simulink model "trjoptmz_MPC_quadcopter1"  (R2024a)
settings: Solver=VariableStepAuto  StartTime=0.0  StopTime=50  FixedStep=0.1  RelTol=1e-3
values from neighbouring files (symbols this model uses):
  g = 9.81    [Quad_innit.m]
  Iz = eye(1)    [Quad_innit.m]
  m = 2    [Quad_innit.m]
  Psi = Psi_temp    [Quad_innit.m]
  Psi_h = Psi_temp    [Quad_innit.m]
  Psi_z = Psi_temp    [Quad_innit.m]
  psid = repmat(psi,ph,1)    [Quad_innit.m]
  Theta = cat(1, Theta, Theta_row)    [Quad_innit.m]
  Theta_h = cat(1, Theta_h, Theta_row)    [Quad_innit.m]
  Theta_z = cat(1, Theta_z, Theta_row)    [Quad_innit.m]
  W3 = (W1.')*W2*W1    [Quad_innit.m]
  W3_h = (W1_h.')*W2_h*W1_h    [Quad_innit.m]
  W3_z = (W1_z.')*W2_z*W1_z    [Quad_innit.m]
  W4 = cat(1, W4, W4_row)    [Quad_innit.m]
  W4_h = cat(1, W4_h, W4_row)    [Quad_innit.m]
  W4_z = cat(1, W4_z, W4_row)    [Quad_innit.m]
libraries: slpidlib x2, sim3dlib x1, uavsim3dlib x1, uavutilslib x1
settings Model: Creator=karthikeyan  LastModifiedBy=karthikeyan

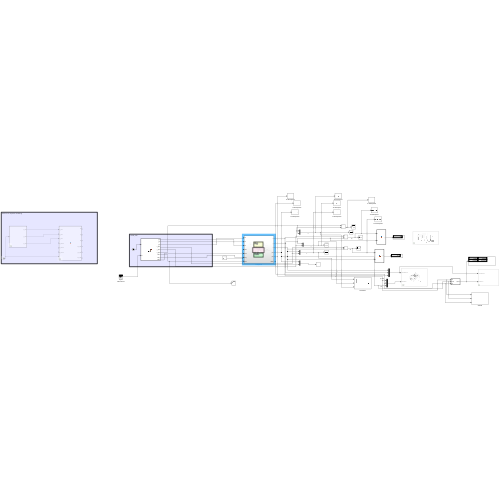
[thumbnail: Simulink's stored preview of the top-level diagram]
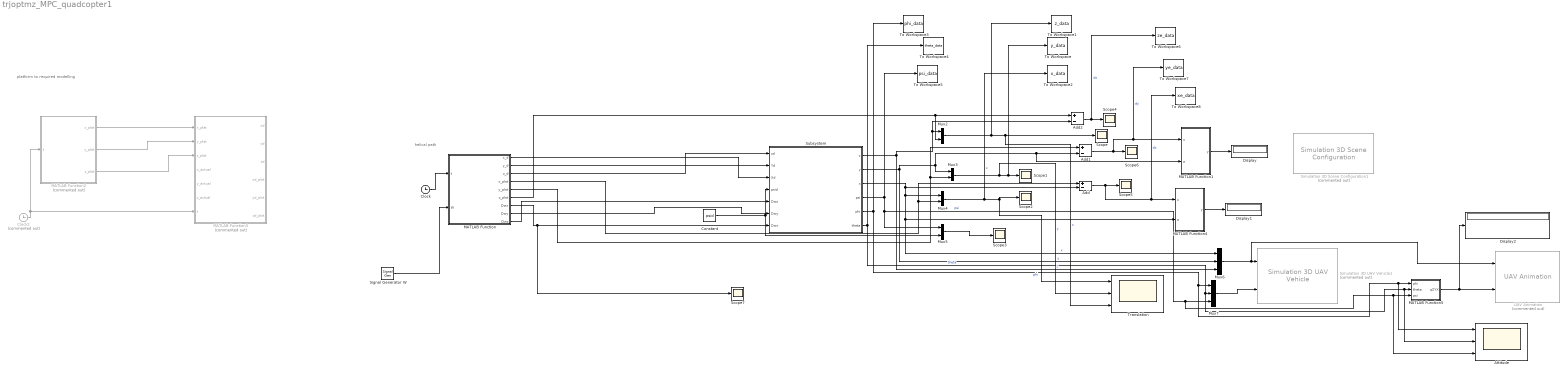
== system trjoptmz_MPC_quadcopter1 ==
  note: platform to required modelling
  note: helical path
  Add : Sum  Inputs=+-
  Add1 : Sum  Inputs=+-
  Add2 : Sum  Inputs=+-
  Attitude : Scope  NumInputPorts=3
  Clock : Clock
  Clock2 : Clock  Commented=on
  Constant : Constant  Value=psid
  Display : Display
  Display1 : Display
  Display2 : Display
  MATLAB Function : MATLAB Function  TreatAsAtomicUnit=on
  MATLAB Function1 : MATLAB Function  TreatAsAtomicUnit=on
  MATLAB Function2 : MATLAB Function  Commented=on  TreatAsAtomicUnit=on
  MATLAB Function3 : MATLAB Function  Commented=on  TreatAsAtomicUnit=on
  MATLAB Function4 : MATLAB Function  TreatAsAtomicUnit=on
  MATLAB Function5 : MATLAB Function  TreatAsAtomicUnit=on
  Mux{2..5} (4 alike) : Mux  Inputs=2
  Mux6 : Mux  Inputs=3
  Mux7 : Mux  Inputs=3
  Scope{,1..7} (8 alike) : Scope
  Signal Generator W : SignalGenerator  WaveForm=random  Units=rad/sec
  Simulation 3D Scene Configuration1 : sim3dlib/Simulation 3D Scene Configuration  Priority=0  Commented=on  ProjectFormat=Default Scenes  SceneDesc=Double lane change  ProjectName=C:\Program Files\MATLAB\R2024a\toolbox\shared\sim3d_projects\automotive_project_windows\UE\WindowsNoEditor\VehicleSimulation.exe  ScenePath=/Game/Maps/EmptyScene  EnableOpenDRIVE=off  vehTagList={'Custom';'Scene Origin';'SimulinkVehicle1';'SimulinkVehicle2'}  vehTag=SimulinkVehicle2  FreeCameraInitialTranslation=[0, 0, 0]  FreeCameraDefaultInitialTranslation=[-6, 0, 2]  FreeCameraInitialRotation=[0, 0, 0]  FreeCameraDefaultInitialRotation=[0, -15, 0]  OpVisEn=off  Ts=0.1  EnableWindow=on  EnableRemoteAccess=off  EnableWeather=off  SunAzimuth=90  SunAltitude=40.0  EnableGeospatialSun=off  Latitude=0  Longitude=0  Date=2023-01-01  Time=10:30:00  GeoTimeZone=-5.0  SunDaylightSaving=off  wind=1  clouds=10  EnableVolumetricClouds=off  CloudCoverage=0  CloudAltitude=6  fog=0  rain=0  RaindropsEffect=off  SnowDensity=0  EnableGeospatial=off  UseTrueOrigin=off  OriginHeight=200  OriginLatitude=40.744652  OriginLongitude=-73.988864  MapStyle=Aerial  AdditionalAssetIDs=[]  UseAdvancedSunSky=off  SolarTime=11  TimeZone=-5  Day=21  Month=9  Year=2022  UseDaylightSavingTime=on  DSTStartDay=10  DSTStartMonth=3  DSTEndDay=3  DSTEndMonth=11  DSTSwitchHour=2  sensorTag=MainCamera2  sensorId=2  sensorName=MainCamera2  mountLoc=Origin  offsetFlag=off  tmountOffset=[0, 0, 0]  rmountOffset=[0, 0, 0]  HorizontalResolution=1280  VerticalResolution=720  HorizontalFOV=60  mountPoint=[0 0 0]  mountOrientation=[0 0 0]  aMode=6  ID=2  GeoTrigger=Inactive
      settings: LibrarySourceBlock=robotsim3dlib/Simulation 3D Scene Configuration
  Simulation 3D UAV Vehicle1 : uavsim3dlib/Simulation 3D UAV Vehicle  Priority=-1  Commented=on  Mesh=Quadrotor  MeshPath=/MathWorksUAVContent/UAVs/HexaRotorUAV/HexaRotor.HexaRotor  Color=Black  ActorName=SimulinkVehicle2  UseGlobalFrame=off  InitialTranslation=[0 0 0]  InitialRotation=[0 0 0]  InitialTranslationGlobal=[0 0 0]  InitialGeoOrigin=[0 0 0]  InitialRotationGlobal=[0 0 0]  SampleTime=-1  ActorType=SimulinkVehicle  ID=2  aMode=4  ActorTag=SimulinkVehicle2
  Subsystem : Subsystem
  To Workspace : ToWorkspace  VariableName=y_data  SaveFormat=Structure With Time  SampleTime=-1
      settings: Save2DSignal=2-D array (concatenate along first dimension)
  To Workspace1 : ToWorkspace  VariableName=z_data  SaveFormat=Structure With Time  SampleTime=-1
      settings: Save2DSignal=2-D array (concatenate along first dimension)
  To Workspace2 : ToWorkspace  VariableName=x_data  SaveFormat=Structure With Time  SampleTime=-1
      settings: Save2DSignal=2-D array (concatenate along first dimension)
  To Workspace3 : ToWorkspace  VariableName=phi_data  SaveFormat=Structure With Time  SampleTime=-1
      settings: Save2DSignal=2-D array (concatenate along first dimension)
  To Workspace4 : ToWorkspace  VariableName=theta_data  SaveFormat=Structure With Time  SampleTime=-1
      settings: Save2DSignal=2-D array (concatenate along first dimension)
  To Workspace5 : ToWorkspace  VariableName=psi_data  SaveFormat=Structure With Time  SampleTime=-1
      settings: Save2DSignal=2-D array (concatenate along first dimension)
  To Workspace6 : ToWorkspace  VariableName=ze_data  SaveFormat=Structure With Time  SampleTime=-1
      settings: Save2DSignal=2-D array (concatenate along first dimension)
  To Workspace7 : ToWorkspace  VariableName=ye_data  SaveFormat=Structure With Time  SampleTime=-1
      settings: Save2DSignal=2-D array (concatenate along first dimension)
  To Workspace8 : ToWorkspace  VariableName=xe_data  SaveFormat=Structure With Time  SampleTime=-1
      settings: Save2DSignal=2-D array (concatenate along first dimension)
  Translation : Scope  NumInputPorts=3
  UAV Animation : uavutilslib/UAV Animation  Commented=on  UAVType=Multirotor  UAVSize=1  InertialZDirection=Up  SampleTime=-1
  wires:
  Subsystem/1(z) -> Add2/2, Mux2/1, Mux6/3  "z"
  Subsystem/2(y) -> Mux3/1, MATLAB Function1/2(a), Add1/2, Mux6/2  "y"
  Subsystem/4(psi) -> To Workspace5/1, Attitude/3, MATLAB Function5/3(psi), Mux7/3, Mux5/1  "psi"
  Mux2/1 -> To Workspace1/1, Translation/3, Scope/1  "z"
  Mux3/1 -> To Workspace/1, Scope1/1, Translation/2  "y"
  MATLAB Function2/2(y_plat) -> MATLAB Function3/2(y_plat)
  MATLAB Function2/3(z_plat) -> MATLAB Function3/3(z_plat)
  Clock2/1 -> MATLAB Function2/1(t), MATLAB Function3/7(t)
  MATLAB Function2/1(x_plat) -> MATLAB Function3/1(x_plat)
  Clock/1 -> MATLAB Function/1(t)
  MATLAB Function/1(x_d) -> Subsystem/3(Xd)
  MATLAB Function/2(y_d) -> Subsystem/2(Yd)
  MATLAB Function/3(z_d) -> Subsystem/1(zd)
  Constant/1 -> Mux5/2, Subsystem/4(psid)
  Mux4/1 -> To Workspace2/1, Scope2/1, Translation/1  "x"
  Mux5/1 -> Scope3/1
  MATLAB Function/4(x_plot) -> Add/1, Mux4/2
  MATLAB Function/5(y_plot) -> Add1/1, Mux3/2
  MATLAB Function/6(z_plot) -> Mux2/2, Add2/1
  Add2/1 -> To Workspace6/1, Scope4/1  "dz"
  Add1/1 -> Scope6/1, To Workspace7/1, MATLAB Function1/1(u)  "dy"
  MATLAB Function1/1(y) -> Display/1
  Subsystem/3(x) -> Mux6/1, MATLAB Function4/2(a), Mux4/1, Add/2  "x"
  MATLAB Function4/1(y) -> Display1/1
  Add/1 -> To Workspace8/1, MATLAB Function4/1(u), Scope5/1  "dx"
  Mux6/1 -> UAV Animation/1, Simulation 3D UAV Vehicle1/1
  Mux7/1 -> Simulation 3D UAV Vehicle1/2
  Subsystem/5(phi) -> To Workspace3/1, Attitude/1, MATLAB Function5/1(phi), Mux7/1  "phi"
  Subsystem/6(theta) -> To Workspace4/1, Attitude/2, MATLAB Function5/2(theta), Mux7/2  "theta"
  MATLAB Function5/1(qZYX) -> Display2/1, UAV Animation/2
  MATLAB Function/7(Dwx) -> Scope7/1, Subsystem/7(Dwx)
  MATLAB Function/8(Dwy) -> Subsystem/6(Dwy)
  MATLAB Function/9(Dwz) -> Subsystem/5(Dwz)
  Signal Generator W/1 -> MATLAB Function/2(W)

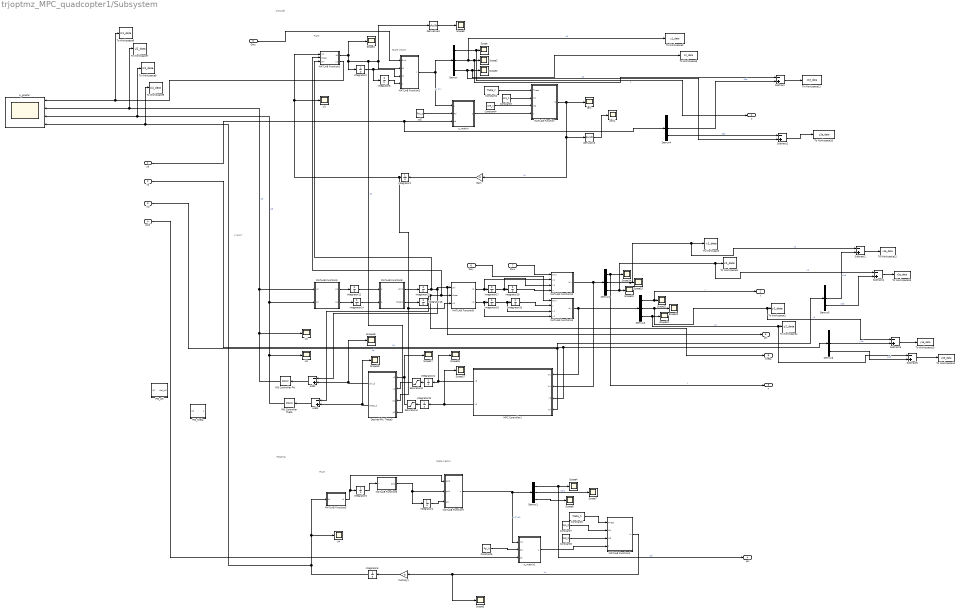
== system trjoptmz_MPC_quadcopter1/Subsystem ==
  note: X and Y
  note: Plant
  note: State Vector
  note: Altitude
  note: State Vector
  note: Plant
  note: Heading
  zd : Inport
  Yd : Inport  Port=2
  Xd : Inport  Port=3
  psid : Inport  Port=4
  Dwz : Inport  Port=5
  Dwy : Inport  Port=6
  Dwx : Inport  Port=7
  Add2 : Sum  Inputs=-+
  Add4 : Sum  Inputs=-+
  Constant2 : Constant  Value=Theta_z
  Constant3 : Constant  Value=W4_z
  Constant4 : Constant  Value=W3_z
  Constant5 : Constant  Value=Psi_h
  Constant6 : Constant  Value=Theta_h
  Constant7 : Constant  Value=W4_h
  Constant8 : Constant  Value=W3_h
  Demux{,1..6} (7 alike) : Demux  Outputs=3
  Derivative : Derivative
  Derivative1 : Derivative
  "Desired Phi, Theta3" : MATLAB Function  TreatAsAtomicUnit=on
  Gain : Gain  Gain=m
  Integrator1 : Integrator  LimitOutput=on  UpperSaturationLimit=1.5*m*g  LowerSaturationLimit=0
  Integrator{12,14..16} (4 alike) : Integrator  WrapState=on
  Integrator17 : Integrator  UpperSaturationLimit=12  LowerSaturationLimit=-12
  Integrator18 : Integrator  LowerSaturationLimit=-12
  Integrator19 : Integrator  UpperSaturationLimit=12  LowerSaturationLimit=-12
  Integrator2 : Integrator  LimitOutput=on  UpperSaturationLimit=10  LowerSaturationLimit=-10  WrappedStateUpperValue=15  WrappedStateLowerValue=-15
  Integrator20 : Integrator  UpperSaturationLimit=12  LowerSaturationLimit=-12
  Integrator21 : Integrator  UpperSaturationLimit=g  LowerSaturationLimit=-g
  Integrator22 : Integrator  UpperSaturationLimit=g  LowerSaturationLimit=-g
  Integrator3 : Integrator
  Integrator4 : Integrator
  Integrator5 : Integrator  UpperSaturationLimit=3.14  LowerSaturationLimit=-3.14  WrapState=on  WrappedStateUpperValue=0.05*1.5*m*g  WrappedStateLowerValue=-0.05*1.5*m*g
  Integrator6 : Integrator  LimitOutput=on  LowerSaturationLimit=0
  MATLAB Function : MATLAB Function  TreatAsAtomicUnit=on
  MATLAB Function1 : MATLAB Function  TreatAsAtomicUnit=on
  MATLAB Function10 : MATLAB Function  TreatAsAtomicUnit=on
  MATLAB Function11 : MATLAB Function  TreatAsAtomicUnit=on
  MATLAB Function2 : MATLAB Function  TreatAsAtomicUnit=on
  MATLAB Function3 : MATLAB Function  TreatAsAtomicUnit=on
  MATLAB Function4 : MATLAB Function  TreatAsAtomicUnit=on
  MATLAB Function5 : MATLAB Function  TreatAsAtomicUnit=on
  MATLAB Function6 : MATLAB Function  TreatAsAtomicUnit=on
  MATLAB Function7 : MATLAB Function  TreatAsAtomicUnit=on
  MATLAB Function8 : MATLAB Function  TreatAsAtomicUnit=on
  MATLAB Function9 : MATLAB Function  TreatAsAtomicUnit=on
  MPC Controller1 : Subsystem
  Multiply1 : Gain  Gain=Iz
  PID Controller Phi : slpidlib/PID Controller  Controller=PID  Form=Parallel  TimeDomain=Continuous-time  UseExternalTs=off  SampleTime=-1  IntegratorMethod=Forward Euler  FilterMethod=Forward Euler  ControllerParametersSource=internal  P=9931.26258398968  I=92443.4670455248  UseKiTs=off  D=250  UseExternalDerivativeSource=off  N=24410.9463918725  UseFilter=on  TunerSelectOption=Transfer Function Based (PID Tuner App)  InitialConditionSource=internal  InitialConditionForIntegrator=0  InitialConditionForFilter=0  DifferentiatorICPrevScaledInput=0  ExternalReset=none  TrackingMode=off  Kt=1  LimitOutput=off  SatLimitsSource=internal  UpperSaturationLimit=inf  LowerSaturationLimit=-inf  LinearizeAsGain=on  AntiWindupMode=none  Kb=1  LimitIntegrator=off  UpperIntegratorSaturationLimit=inf  LowerIntegratorSaturationLimit=-inf  POutMin=[]  POutMax=[]  IOutMin=[]  IOutMax=[]  DOutMin=[]  DOutMax=[]  NOutMin=[]  NOutMax=[]  SumOutMin=[]  SumOutMax=[]  SaturationOutMin=[]  SaturationOutMax=[]  PParamMin=[]  PParamMax=[]  IParamMin=[]  IParamMax=[]  DParamMin=[]  DParamMax=[]  NParamMin=[]  NParamMax=[]  KbParamMin=[]  KbParamMax=[]  KtParamMin=[]  KtParamMax=[]  KbOutMin=[]  KbOutMax=[]  KtOutMin=[]  KtOutMax=[]  IntegratorOutMin=[]  IntegratorOutMax=[]  FilterOutMin=[]  FilterOutMax=[]  SumI1OutMin=[]  SumI1OutMax=[]  SumI2OutMin=[]  SumI2OutMax=[]  SumI3OutMin=[]  SumI3OutMax=[]  SumI4OutMin=[]  SumI4OutMax=[]  SumDOutMin=[]  SumDOutMax=[]  DifferentiatorOutMin=[]  DifferentiatorOutMax=[]  FilterDiffOutCoefMin=[]  FilterDiffOutCoefMax=[]  ReciprocalOutMin=[]  ReciprocalOutMax=[]  SumDenOutMin=[]  SumDenOutMax=[]  SumNumOutMin=[]  SumNumOutMax=[]  DivideOutMin=[]  DivideOutMax=[]  UdiffTsProdOutMin=[]  UdiffTsProdOutMax=[]  NTsProdOutMin=[]  NTsProdOutMax=[]  UintegralTsProdOutMin=[]  UintegralTsProdOutMax=[]  UngainTsProdOutMin=[]  UngainTsProdOutMax=[]  ClampingZeroOutDataTypeStr=Inherit: Inherit via back propagation  ClampingZeroOutMin=[]  ClampingZeroOutMax=[]  FilterDenConstantOutDataTypeStr=Inherit: Inherit via back propagation  FilterDenConstantOutMin=[]  FilterDenConstantOutMax=[]  PCopyOutDataTypeStr=Inherit: Inherit via back propagation  PCopyOutMin=[]  PCopyOutMax=[]  NCopyOutDataTypeStr=Inherit: Inherit via back propagation  NCopyOutMin=[]  NCopyOutMax=[]  IntegratorContinuousStateAttributes=''  IntegratorStateMustResolveToSignalObject=off  IntegratorRTWStateStorageClass=Auto  FilterContinuousStateAttributes=''  FilterStateMustResolveToSignalObject=off  FilterRTWStateStorageClass=Auto  ParallelPVariant=InternalParameters  IdealPVariant=Disabled  IVariant=InternalParameters  DVariant=InternalParameters  IntegratorVariant=Continuous  SatVariant=Disabled  AWVariant=Passthrough  PCopyVariant=Disabled  TRVariant=Disabled  FdbkBlocksVariant=Forward  IdealPFdbkVariant=Disabled  SatFdbkVariant=Disabled  DerivativeFilterVariant=ContFilter  NVariant=InternalParameters  NCopyVariant=Disabled  FilterICVariant=InternalICsFilter  IntegratorICVariant=InternalICs  ExternalResetVariant=Disabled  TRSumVariant=Passthrough  SumFdbkVariant=Disabled  SumVariant=Sum_PID  TsampFilterVariant=InternalTs  TsampNgainVariant=Passthrough  TsampIntegralVariant=Disabled_SignalSpec  ExternalSaturationOutDataTypeStr=Inherit: Same as second input  DerivativeSourceVariant=ErrorSignal
  PID Controller Theta : slpidlib/PID Controller  Controller=PID  Form=Parallel  TimeDomain=Continuous-time  UseExternalTs=off  SampleTime=-1  IntegratorMethod=Forward Euler  FilterMethod=Forward Euler  ControllerParametersSource=internal  P=10811.4487421448  I=110533.695685683  UseKiTs=off  D=250  UseExternalDerivativeSource=off  N=24410.9463914125  UseFilter=on  TunerSelectOption=Transfer Function Based (PID Tuner App)  InitialConditionSource=internal  InitialConditionForIntegrator=0  InitialConditionForFilter=0  DifferentiatorICPrevScaledInput=0  ExternalReset=none  TrackingMode=off  Kt=1  LimitOutput=off  SatLimitsSource=internal  UpperSaturationLimit=inf  LowerSaturationLimit=-inf  LinearizeAsGain=on  AntiWindupMode=none  Kb=1  LimitIntegrator=off  UpperIntegratorSaturationLimit=inf  LowerIntegratorSaturationLimit=-inf  POutMin=[]  POutMax=[]  IOutMin=[]  IOutMax=[]  DOutMin=[]  DOutMax=[]  NOutMin=[]  NOutMax=[]  SumOutMin=[]  SumOutMax=[]  SaturationOutMin=[]  SaturationOutMax=[]  PParamMin=[]  PParamMax=[]  IParamMin=[]  IParamMax=[]  DParamMin=[]  DParamMax=[]  NParamMin=[]  NParamMax=[]  KbParamMin=[]  KbParamMax=[]  KtParamMin=[]  KtParamMax=[]  KbOutMin=[]  KbOutMax=[]  KtOutMin=[]  KtOutMax=[]  IntegratorOutMin=[]  IntegratorOutMax=[]  FilterOutMin=[]  FilterOutMax=[]  SumI1OutMin=[]  SumI1OutMax=[]  SumI2OutMin=[]  SumI2OutMax=[]  SumI3OutMin=[]  SumI3OutMax=[]  SumI4OutMin=[]  SumI4OutMax=[]  SumDOutMin=[]  SumDOutMax=[]  DifferentiatorOutMin=[]  DifferentiatorOutMax=[]  FilterDiffOutCoefMin=[]  FilterDiffOutCoefMax=[]  ReciprocalOutMin=[]  ReciprocalOutMax=[]  SumDenOutMin=[]  SumDenOutMax=[]  SumNumOutMin=[]  SumNumOutMax=[]  DivideOutMin=[]  DivideOutMax=[]  UdiffTsProdOutMin=[]  UdiffTsProdOutMax=[]  NTsProdOutMin=[]  NTsProdOutMax=[]  UintegralTsProdOutMin=[]  UintegralTsProdOutMax=[]  UngainTsProdOutMin=[]  UngainTsProdOutMax=[]  ClampingZeroOutDataTypeStr=Inherit: Inherit via back propagation  ClampingZeroOutMin=[]  ClampingZeroOutMax=[]  FilterDenConstantOutDataTypeStr=Inherit: Inherit via back propagation  FilterDenConstantOutMin=[]  FilterDenConstantOutMax=[]  PCopyOutDataTypeStr=Inherit: Inherit via back propagation  PCopyOutMin=[]  PCopyOutMax=[]  NCopyOutDataTypeStr=Inherit: Inherit via back propagation  NCopyOutMin=[]  NCopyOutMax=[]  IntegratorContinuousStateAttributes=''  IntegratorStateMustResolveToSignalObject=off  IntegratorRTWStateStorageClass=Auto  FilterContinuousStateAttributes=''  FilterStateMustResolveToSignalObject=off  FilterRTWStateStorageClass=Auto  ParallelPVariant=InternalParameters  IdealPVariant=Disabled  IVariant=InternalParameters  DVariant=InternalParameters  IntegratorVariant=Continuous  SatVariant=Disabled  AWVariant=Passthrough  PCopyVariant=Disabled  TRVariant=Disabled  FdbkBlocksVariant=Forward  IdealPFdbkVariant=Disabled  SatFdbkVariant=Disabled  DerivativeFilterVariant=ContFilter  NVariant=InternalParameters  NCopyVariant=Disabled  FilterICVariant=InternalICsFilter  IntegratorICVariant=InternalICs  ExternalResetVariant=Disabled  TRSumVariant=Passthrough  SumFdbkVariant=Disabled  SumVariant=Sum_PID  TsampFilterVariant=InternalTs  TsampNgainVariant=Passthrough  TsampIntegralVariant=Disabled_SignalSpec  ExternalSaturationOutDataTypeStr=Inherit: Same as second input  DerivativeSourceVariant=ErrorSignal
  PID_phi : Subsystem
  PID_theta : Subsystem
  Saturation3 : Saturate  UpperLimit=1  LowerLimit=-1
  Saturation4 : Saturate  UpperLimit=1  LowerLimit=-1
  Scope{,1..5,7..9,14..15,17..23,26..27} (20 alike) : Scope
  Subtract{,1..5} (6 alike) : Sum  Inputs=-+
  To Workspace : ToWorkspace  VariableName=x1_data  SaveFormat=Structure With Time  SampleTime=-1
      settings: Save2DSignal=2-D array (concatenate along first dimension)
  To Workspace1 : ToWorkspace  VariableName=y1_data  SaveFormat=Structure With Time  SampleTime=-1
      settings: Save2DSignal=2-D array (concatenate along first dimension)
  To Workspace10 : ToWorkspace  VariableName=z2e_data  SaveFormat=Structure With Time  SampleTime=-1
      settings: Save2DSignal=2-D array (concatenate along first dimension)
  To Workspace11 : ToWorkspace  VariableName=z1e_data  SaveFormat=Structure With Time  SampleTime=-1
      settings: Save2DSignal=2-D array (concatenate along first dimension)
  To Workspace12 : ToWorkspace  VariableName=x1e_data  SaveFormat=Structure With Time  SampleTime=-1
      settings: Save2DSignal=2-D array (concatenate along first dimension)
  To Workspace13 : ToWorkspace  VariableName=x2e_data  SaveFormat=Structure With Time  SampleTime=-1
      settings: Save2DSignal=2-D array (concatenate along first dimension)
  To Workspace14 : ToWorkspace  VariableName=y2e_data  SaveFormat=Structure With Time  SampleTime=-1
      settings: Save2DSignal=2-D array (concatenate along first dimension)
  To Workspace15 : ToWorkspace  VariableName=y1e_data  SaveFormat=Structure With Time  SampleTime=-1
      settings: Save2DSignal=2-D array (concatenate along first dimension)
  To Workspace2 : ToWorkspace  VariableName=z1_data  SaveFormat=Structure With Time  SampleTime=-1
      settings: Save2DSignal=2-D array (concatenate along first dimension)
  To Workspace3 : ToWorkspace  VariableName=x2_data  SaveFormat=Structure With Time  SampleTime=-1
      settings: Save2DSignal=2-D array (concatenate along first dimension)
  To Workspace4 : ToWorkspace  VariableName=y2_data  SaveFormat=Structure With Time  SampleTime=-1
      settings: Save2DSignal=2-D array (concatenate along first dimension)
  To Workspace5 : ToWorkspace  VariableName=z2_data  SaveFormat=Structure With Time  SampleTime=-1
      settings: Save2DSignal=2-D array (concatenate along first dimension)
  To Workspace6 : ToWorkspace  VariableName=U1_data  SaveFormat=Structure With Time  SampleTime=-1
      settings: Save2DSignal=2-D array (concatenate along first dimension)
  To Workspace7 : ToWorkspace  VariableName=U2_data  SaveFormat=Structure With Time  SampleTime=-1
      settings: Save2DSignal=2-D array (concatenate along first dimension)
  To Workspace8 : ToWorkspace  VariableName=U3_data  SaveFormat=Structure With Time  SampleTime=-1
      settings: Save2DSignal=2-D array (concatenate along first dimension)
  To Workspace9 : ToWorkspace  VariableName=U4_data  SaveFormat=Structure With Time  SampleTime=-1
      settings: Save2DSignal=2-D array (concatenate along first dimension)
  U{1..4} (4 alike) : Scope
  U_graphs : Scope  NumInputPorts=4
  jerk : Scope
  jerk1 : Scope
  s_matrix : MATLAB Function  TreatAsAtomicUnit=on
  s_matrix1 : MATLAB Function  TreatAsAtomicUnit=on
  zd2 : Constant  Value=Psi_z
  z : Outport
  y : Outport  Port=2
  x : Outport  Port=3
  psi : Outport  Port=4
  phi : Outport  Port=5
  theta : Outport  Port=6
  wires:
  Integrator3/1 -> MATLAB Function6/1(r)
  Integrator14/1 -> MATLAB Function8/2(q)
  MATLAB Function3/2(q1) -> Integrator14/1
  Derivative1/1 -> Scope9/1
  PID Controller Phi/1 -> To Workspace7/1, U_graphs/2, MATLAB Function3/1(u2), U2/1  "U2"
  Integrator4/1 -> MATLAB Function7/3(psi)
  Integrator6/1 -> MATLAB Function2/4(z)
  Demux2/1 -> x/1, Scope14/1  "x"
  "Desired Phi, Theta3"/1(phi_d) -> Add2/2, Scope18/1
  Integrator19/1 -> MATLAB Function10/4(x)
  Multiply1/1 -> Integrator5/1
  Integrator16/1 -> Add4/1, theta/1, MATLAB Function1/2(theta), MATLAB Function9/2(theta)
  Demux1/1 -> psi/1, Scope4/1  "psi"
  MATLAB Function1/1(z2) -> "Desired Phi, Theta3"/4(z2), Derivative1/1, MATLAB Function2/2(z2), Integrator2/1, Scope1/1  "z2"
  Constant3/1 -> MATLAB Function/2(W4)
  Integrator2/1 -> MATLAB Function2/3(z1), Integrator6/1
  Demux/3 -> Subtract1/2, To Workspace5/1, Scope3/1  "z2"
  MATLAB Function6/1(psi1) -> Integrator4/1, MATLAB Function7/2(psi1)
  Add4/1 -> PID Controller Theta/1
  Demux3/1 -> y/1, Scope21/1  "y"
  MATLAB Function4/1(vk) -> Scope5/1, Multiply1/1  "Vk"
  Integrator5/1 -> To Workspace9/1, U_graphs/4, MATLAB Function5/1(U4), U4/1
  s_matrix/1(s) -> MATLAB Function/4(s)
  Integrator17/1 -> MATLAB Function10/3(x1), Integrator19/1
  Integrator21/1 -> Saturation3/1
  Integrator15/1 -> MATLAB Function1/3(phi), Add2/1, phi/1, MATLAB Function9/1(phi)
  MATLAB Function/1(vk) -> Gain/1, Derivative/1, jerk/1  "Vk"
  Gain/1 -> Integrator1/1
  MATLAB Function5/1(r1) -> Integrator3/1, MATLAB Function7/1(psi2)
  Add2/1 -> PID Controller Phi/1
  Demux/1 -> z/1, Scope/1  "z"
  PID Controller Theta/1 -> To Workspace8/1, U_graphs/3, MATLAB Function3/2(u3), U3/1  "U3"
  MATLAB Function7/1(w) -> Demux1/1, s_matrix1/1(Wk)  "z = Wk"
  Integrator18/1 -> MATLAB Function11/3(y1), Integrator20/1
  zd2/1 -> s_matrix/2(Psi)
  MATLAB Function9/2(y2) -> MATLAB Function11/4(y2), Integrator18/1
  Integrator1/1 -> MATLAB Function9/3(U1), "Desired Phi, Theta3"/3(U1), MATLAB Function1/1(U1), U1/1
  "Desired Phi, Theta3"/2(theta_d) -> Scope19/1, Add4/2
  Derivative/1 -> jerk1/1
  Constant2/1 -> MATLAB Function/1(Theta)
  Saturation4/1 -> Scope17/1, "Desired Phi, Theta3"/1(x2)
  Constant7/1 -> MATLAB Function4/2(W4)
  Constant5/1 -> s_matrix1/2(Psi)
  Integrator20/1 -> MATLAB Function11/2(y)
  Constant8/1 -> MATLAB Function4/3(W3)
  Demux1/3 -> Scope8/1
  Demux2/3 -> Subtract4/1, To Workspace3/1, Scope20/1  "x2"
  psid/1 -> s_matrix1/3(zd)
  Demux2/2 -> Subtract2/1, To Workspace/1, Scope15/1  "x1"
  Demux1/2 -> Scope7/1  "psi1"
  Constant4/1 -> MATLAB Function/3(W3)
  MATLAB Function3/1(p1) -> Integrator12/1
  MATLAB Function8/2(theta1) -> Integrator16/1
  Demux/2 -> To Workspace2/1, Subtract/1, Scope2/1  "z1"
  MATLAB Function10/1(Wx) -> Demux2/1, MPC Controller1/2(Wx)
  MATLAB Function8/1(phi1) -> Integrator15/1
  Demux3/2 -> Subtract3/1, To Workspace1/1, Scope22/1  "y1"
  Demux3/3 -> Subtract5/1, To Workspace4/1, Scope23/1  "y2"
  MATLAB Function11/1(Wy) -> MPC Controller1/1(Wy), Demux3/1
  Integrator12/1 -> MATLAB Function8/1(p)
  MPC Controller1/1(y3) -> Integrator21/1, Scope26/1
  MATLAB Function2/1(x) -> s_matrix/1(x), Demux/1  "y = x"
  MATLAB Function9/1(x2) -> MATLAB Function10/2(x2), Integrator17/1
  MPC Controller1/2(x3) -> Scope27/1, Integrator22/1
  Saturation3/1 -> "Desired Phi, Theta3"/2(y2)
  Integrator22/1 -> Saturation4/1
  Constant6/1 -> MATLAB Function4/1(Theta)
  s_matrix1/1(s) -> MATLAB Function4/4(s)
  Xd/1 -> Demux5/1, MPC Controller1/4(Xd)  "Xd"
  zd/1 -> Demux4/1, s_matrix/3(zd)
  Yd/1 -> Demux6/1, MPC Controller1/3(Yd)  "Yd"
  MATLAB Function1/2(u1) -> To Workspace6/1, U_graphs/1
  Dwz/1 -> MATLAB Function2/1(Dwz)
  Dwx/1 -> MATLAB Function10/1(Dwx)
  Dwy/1 -> MATLAB Function11/1(Dwx)
  Demux4/2 -> Subtract/2  "z1d"
  Demux4/3 -> Subtract1/1  "z2d"
  Subtract/1 -> To Workspace11/1
  Subtract1/1 -> To Workspace10/1
  Demux5/2 -> Subtract2/2  "x1d"
  Demux5/3 -> Subtract4/2  "x2d"
  Demux6/2 -> Subtract3/2  "y1d"
  Demux6/3 -> Subtract5/2  "y2d"
  Subtract2/1 -> To Workspace12/1
  Subtract4/1 -> To Workspace13/1
  Subtract5/1 -> To Workspace14/1
  Subtract3/1 -> To Workspace15/1

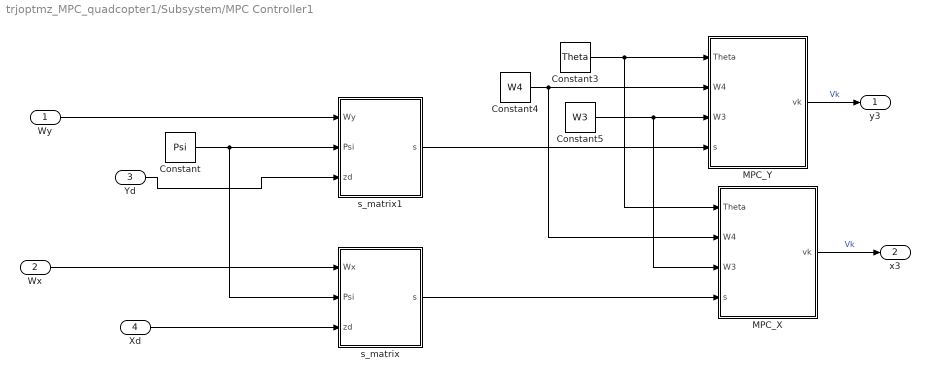
== system trjoptmz_MPC_quadcopter1/Subsystem/MPC Controller1 ==
  Wy : Inport
  Wx : Inport  Port=2
  Yd : Inport  Port=3
  Xd : Inport  Port=4
  Constant : Constant  Value=Psi
  Constant3 : Constant  Value=Theta
  Constant4 : Constant  Value=W4
  Constant5 : Constant  Value=W3
  MPC_X : MATLAB Function  TreatAsAtomicUnit=on
  MPC_Y : MATLAB Function  TreatAsAtomicUnit=on
  s_matrix : MATLAB Function  TreatAsAtomicUnit=on
  s_matrix1 : MATLAB Function  TreatAsAtomicUnit=on
  y3 : Outport
  x3 : Outport  Port=2
  wires:
  Constant3/1 -> MPC_Y/1(Theta), MPC_X/1(Theta)
  Constant/1 -> s_matrix1/2(Psi), s_matrix/2(Psi)
  Constant4/1 -> MPC_Y/2(W4), MPC_X/2(W4)
  Constant5/1 -> MPC_Y/3(W3), MPC_X/3(W3)
  s_matrix1/1(s) -> MPC_Y/4(s)
  s_matrix/1(s) -> MPC_X/4(s)
  Xd/1 -> s_matrix/3(zd)
  Yd/1 -> s_matrix1/3(zd)
  MPC_Y/1(vk) -> y3/1  "Vk"
  MPC_X/1(vk) -> x3/1  "Vk"
  Wx/1 -> s_matrix/1(Wx)
  Wy/1 -> s_matrix1/1(Wy)

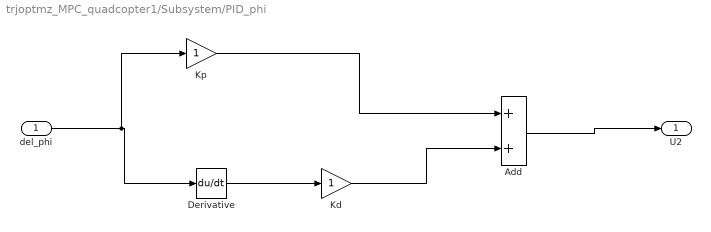
== system trjoptmz_MPC_quadcopter1/Subsystem/PID_phi ==
  del_phi : Inport
  Add : Sum
  Derivative : Derivative
  Kd : Gain
  Kp : Gain
  U2 : Outport
  wires:
  del_phi/1 -> Derivative/1, Kp/1
  Derivative/1 -> Kd/1
  Kp/1 -> Add/1
  Add/1 -> U2/1
  Kd/1 -> Add/2

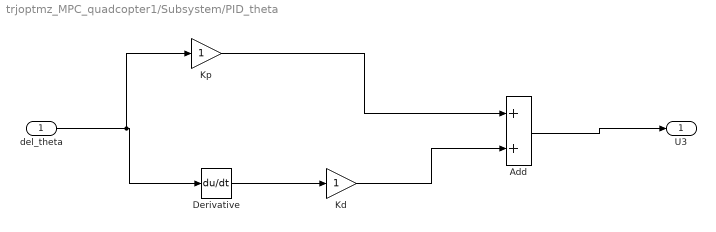
== system trjoptmz_MPC_quadcopter1/Subsystem/PID_theta ==
  del_theta : Inport
  Add : Sum
  Derivative : Derivative
  Kd : Gain
  Kp : Gain
  U3 : Outport
  wires:
  del_theta/1 -> Derivative/1, Kp/1
  Derivative/1 -> Kd/1
  Kp/1 -> Add/1
  Add/1 -> U3/1
  Kd/1 -> Add/2

== matlab function trjoptmz_MPC_quadcopter1/Subsystem/s_matrix1 ==
  data: Wk input; Psi input; zd input; s output
function s = fcn(Wk,Psi,zd)
% zk = C1*Wk;
s = zd-(Psi*Wk);

== matlab function trjoptmz_MPC_quadcopter1/MATLAB Function ==
  data: t input; x_d output; y_d output; z_d output; x_plot output; y_plot output; z_plot output; Dwx output; Dwy output; Dwz output; W input
function [x_d, y_d, z_d, x_plot, y_plot, z_plot, Dwx, Dwy, Dwz]= trajectory(t,W)


R = 2;
w = 0.1*3.14;
p = 5;
pz = 5;
h = 0.5;
del_t = 0.01;
%% Circular spiral Trajectory
% x_func = @(u) R*sin(u*w);
% y_func = @(u) R - r(u)*cos(u*w);
% z_func = @(u) 0.5*u;
% 
% x_v_func = @(u) R*w*(cos(u*w));
% y_v_func = @(u) R*w*(sin(u*w));
% z_v_func = @(u) 0.5;
% 
% x_a_func = @(u) -R*w^2 *(sin(u*w));%-r*w^2 *sin(u*w);
% y_a_func = @(u) R*w^2 *(cos(u*w));
% z_a_func = @(u) 0;

%% Conical spiral Trajectory
r = @(u) u*pi/100;
x_func = @(u) r(u)*cos(u*w);
y_func = @(u) r(u)*sin(u*w);
z_func = @(u) 0.5*u;

x_v_func = @(u) -r(u)*w*(sin(u*w));
y_v_func = @(u) r(u)*w*(cos(u*w));
z_v_func = @(u) 0.5;

x_a_func = @(u) -r(u)*w^2 *(cos(u*w));%-r*w^2 *sin(u*w);
y_a_func = @(u) -r(u)*w^2 *(sin(u*w));
z_a_func = @(u) 0;
%% Climb and track 8


dwx =@(u) (2*sin(W*pi*u));
dwy =@(u) -1*sin(W*pi*u);
dwz =@(u) 0.8*sin(W*pi*u);

xd = zeros(p*3, 1);
yd = zeros(p*3, 1);
zd = zeros(p*3, 1);


flag = 1;
for i = 0:p-1
    xd(flag) = x_func(t + i*del_t);
    xd(flag + 1) = x_v_func(t + i*del_t);
    xd(flag + 2) = x_a_func(t+ i*del_t);

    yd(flag ) = y_func(t+ i*del_t);
    yd(flag + 1) = y_v_func(t+ i*del_t);
    yd(flag +2) = y_a_func(t+ i*del_t);

    zd(flag  ) = z_func(t+ i*del_t);
    zd(flag + 1) = z_v_func(t+ i*del_t);
    zd(flag + 2) = z_a_func(t+ i*del_t);

    flag = flag + 3;


end

x_d = xd;
y_d = yd;
z_d = zd;

x_plot = xd(1);
y_plot = yd(1);
z_plot = zd(1);

Dwx = 0; %dwx(t);
Dwy = 0; %dwy(t);
Dwz = 0; %dwz(t);

== matlab function trjoptmz_MPC_quadcopter1/MATLAB Function2 ==
  data: t input; x_plat output; y_plat output; z_plat output
function [x_plat, y_plat, z_plat] = platform_trajectory(t)





r = 5;
w = 3;


x_plat = 3;
y_plat = 4;
z_plat = 0;

== matlab function trjoptmz_MPC_quadcopter1/Subsystem/Desired Phi, Theta3 ==
  data: x2 input; phi_d output; y2 input; theta_d output; U1 input; z2 input
function [phi_d,theta_d] = fcn(x2,y2,U1,z2)
m = 2; g = 9.81; 
U1 = m*g; z2 = 0; % Hover condition
if U1 == 0
    U1 = 1e-3;
end
if z2 == -g
    z2 = z2+(1e-3);
end
theta_d = asin((-m*x2/U1));
phi_d = atan(cos(theta_d)*y2/(z2+g));

== matlab function trjoptmz_MPC_quadcopter1/Subsystem/MATLAB Function3 ==
  data: u2 input; p1 output; u3 input; q1 output
function [p1,q1] = fcn(u2,u3)
Ix = 1.25; Iy = 1.25;

p1 = u2/Ix;
q1 = u3/Iy;

== matlab function trjoptmz_MPC_quadcopter1/Subsystem/MATLAB Function8 ==
  data: p input; phi1 output; q input; theta1 output
function [phi1,theta1] = fcn(p,q)

phi1 = p;
theta1 = q;

== matlab function trjoptmz_MPC_quadcopter1/Subsystem/MATLAB Function9 ==
  data: phi input; x2 output; theta input; y2 output; U1 input
function [x2,y2] = fcn(phi,theta,U1)
m = 2; g = 9.81;
%U1 = m*g;  % Hover condition

x2 = -sin(theta)*U1/m;
y2 = sin(phi)*cos(theta)*U1/m;

== matlab function trjoptmz_MPC_quadcopter1/Subsystem/MATLAB Function10 ==
  data: Dwx input; x2 input; x1 input; x input; Wx output
function Wx = fcn(Dwx,x2,x1,x)

Wx = [x;x1;(x2+Dwx)];

== matlab function trjoptmz_MPC_quadcopter1/Subsystem/MATLAB Function11 ==
  data: Dwx input; y input; Wy output; y1 input; y2 input
function Wy = fcn(Dwx,y,y1,y2)

Wy = [y;y1;(y2+Dwx)];

== matlab function trjoptmz_MPC_quadcopter1/Subsystem/MPC Controller1/MPC_X ==
  data: Theta input; vk output; W4 input; W3 input; s input
function vk = fcn(Theta,W4,W3,s)
T = Theta.';

v = (inv((T*W4*Theta)+W3))*(T)*W4*s;
vk = v(1);

== matlab function trjoptmz_MPC_quadcopter1/Subsystem/MPC Controller1/MPC_Y ==
  data: Theta input; vk output; W4 input; W3 input; s input
function vk = fcn(Theta,W4,W3,s)
T = Theta.';

v = (inv((T*W4*Theta)+W3))*(T)*W4*s;
vk = v(1);

== matlab function trjoptmz_MPC_quadcopter1/Subsystem/MPC Controller1/s_matrix ==
  data: Wx input; Psi input; zd input; s output
function s = fcn(Wx,Psi,zd)

s = zd-(Psi*Wx);

== matlab function trjoptmz_MPC_quadcopter1/Subsystem/MPC Controller1/s_matrix1 ==
  data: Wy input; Psi input; zd input; s output
function s = fcn(Wy,Psi,zd)

s = zd-(Psi*Wy);

== matlab function trjoptmz_MPC_quadcopter1/Subsystem/MATLAB Function ==
  data: Theta input; vk output; W4 input; W3 input; s input
function vk = fcn(Theta,W4,W3,s)
T = Theta.';

v = (inv((T*W4*Theta)+W3))*(T)*W4*s;
vk = v(1);

== matlab function trjoptmz_MPC_quadcopter1/MATLAB Function3 ==
  data: x_plat input; xd output; yd output; zd output; y_plat input; z_plat input; xd_plot output; yd_plot output; zd_plot output; x_actual input; y_actual input; z_actual input; t input
function [xd, yd, zd, xd_plot, yd_plot, zd_plot] = trajectory(x_plat,y_plat,z_plat, x_actual, y_actual, z_actual, t)


p = 5;
h = 0.1;


if z_actual <= 10
    zd = repmat([10; 0 ; 0], p, 1);
    xd = repmat([x_actual; 0 ; 0], p , 1);
    yd = repmat([y_actual; 0 ; 0], p, 1);

    if((x_plat - x_actual) < ERROR && (y_plat - y_actual) < ERROR)
    
    z_traj = 0;
    zd = repmat([z_traj; 0 ; 0], p, 1);
    else
    xd = repmat([x_plat; 0 ; 0], p, 1);
    yd = repmat([y_plat; 0;0], p, 1);

    end
else
    zd = repmat([10; 0 ; 0], p, 1);
    xd = repmat([x_plat; 0 ; 0], p , 1);
    yd = repmat([y_plat; 0 ; 0], p, 1);
end 



zd_plot = zd(1);
yd_plot = yd(1);
xd_plot = xd(1);

== matlab function trjoptmz_MPC_quadcopter1/MATLAB Function1 ==
  data: u input; y output; a input
function y = fcn(u,a)

y = u*100/a;

== matlab function trjoptmz_MPC_quadcopter1/MATLAB Function4 ==
  data: u input; y output; a input
function y = fcn(u,a)

y = u*100/a;

== matlab function trjoptmz_MPC_quadcopter1/Subsystem/s_matrix ==
  data: x input; Psi input; zd input; s output
function s = fcn(x,Psi,zd)

s = zd-(Psi*x);

== matlab function trjoptmz_MPC_quadcopter1/Subsystem/MATLAB Function1 ==
  data: U1 input; z2 output; theta input; phi input; u1 output
function [z2,u1] = fcn(U1,theta, phi)

%phi = 0; theta = 0; 
g = 9.81; m = 2;
u1 = U1/(cos(phi)*cos(theta));
z2 = (cos(phi)*cos(theta)*u1/m)-g;

== matlab function trjoptmz_MPC_quadcopter1/Subsystem/MATLAB Function2 ==
  data: Dwz input; z2 input; x output; z1 input; z input
function x = fcn(Dwz,z2,z1,z)

x = [z;z1;(z2+Dwz)];

== matlab function trjoptmz_MPC_quadcopter1/MATLAB Function5 ==
  data: phi input; qZYX output; theta input; psi input
function qZYX = fcn(phi,theta,psi)

eul = [psi theta phi];
qZYX = eul2quat(eul);

== matlab function trjoptmz_MPC_quadcopter1/Subsystem/MATLAB Function4 ==
  data: Theta input; vk output; W4 input; W3 input; s input
function vk = fcn(Theta,W4,W3,s)
T = Theta.';

v = (inv((T*W4*Theta)+W3))*(T)*W4*s;
vk = v(1);

== matlab function trjoptmz_MPC_quadcopter1/Subsystem/MATLAB Function5 ==
  data: U4 input; r1 output
function r1 = fcn(U4)
Iz = 2.5;
r1 = U4/Iz;

== matlab function trjoptmz_MPC_quadcopter1/Subsystem/MATLAB Function6 ==
  data: r input; psi1 output
function psi1 = fcn(r)

psi1 = r;

== matlab function trjoptmz_MPC_quadcopter1/Subsystem/MATLAB Function7 ==
  data: psi2 input; psi1 input; psi input; w output
function w = fcn(psi2,psi1,psi)
% psi2 = r1
w = [psi;psi1;psi2];
size(w);
